simulink model "exer2"  (R2012b)
settings: Solver=ode45  StartTime=0.0  StopTime=10.0  RelTol=1e-3
undefined symbols (not defined in the file): alfa, epson, omega

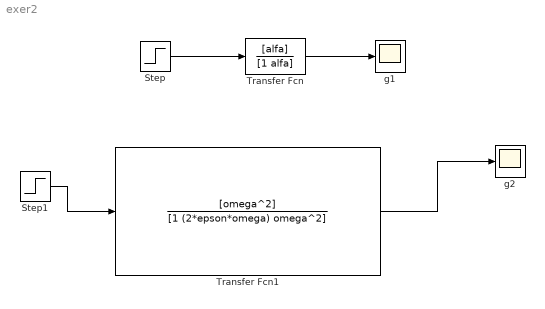
== system exer2 ==
  Step : Step  SampleTime=0
  Step1 : Step  SampleTime=0
  Transfer Fcn : TransferFcn  Numerator=[alfa]  Denominator=[1 alfa]
  Transfer Fcn1 : TransferFcn  Numerator=[omega^2]  Denominator=[1 (2*epson*omega) omega^2]
  g1 : Scope
  g2 : Scope
  wires:
  Step/1 -> Transfer Fcn/1
  Transfer Fcn/1 -> g1/1
  Step1/1 -> Transfer Fcn1/1
  Transfer Fcn1/1 -> g2/1
